simulink model "positioning_system"  (R2021a)
settings: Solver=ode45  StartTime=0.0  StopTime=2  RelTol=1e-3
values from neighbouring files (symbols this model uses):
  C = 0.33*(10^-6)    (= 3.3e-07)    [run_positioning_system.m]
  d = 1    [run_positioning_system.m]
  Km = 5*(10^-3)    (= 0.005)    [run_positioning_system.m]
  Ks = 52.5    [run_positioning_system.m]
  P = 60000    [run_positioning_system.m]
  R = 10000    [run_positioning_system.m]
settings Model: Creator=sujit  LastModifiedBy=cop20skj
settings SolverCC: AlgebraicLoopSolver=TrustRegion
settings DataIOCC: ReturnWorkspaceOutputs=off
settings DebuggingCC: SFMachineParentedDataDiag=warning

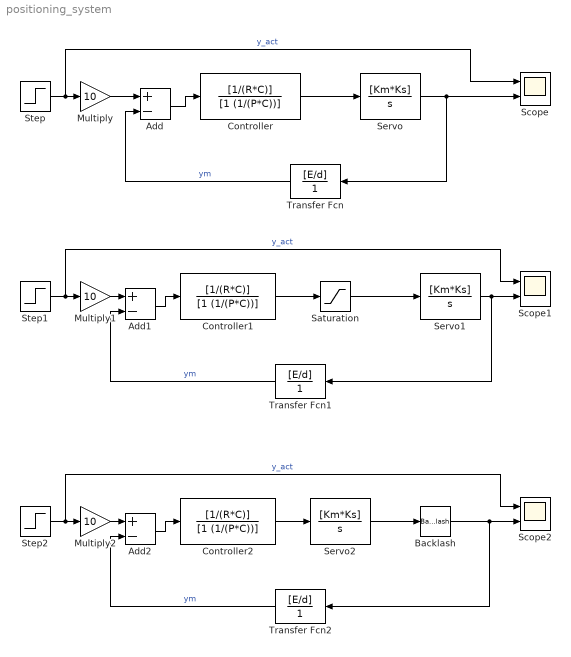
== system positioning_system ==
  Add : Sum  Inputs=+-
  Add1 : Sum  Inputs=+-
  Add2 : Sum  Inputs=+-
  Backlash : Backlash
  Controller : TransferFcn  Numerator=[1/(R*C)]  Denominator=[1 (1/(P*C))]
  Controller1 : TransferFcn  Numerator=[1/(R*C)]  Denominator=[1 (1/(P*C))]
  Controller2 : TransferFcn  Numerator=[1/(R*C)]  Denominator=[1 (1/(P*C))]
  Multiply : Gain  Gain=10
  Multiply1 : Gain  Gain=10
  Multiply2 : Gain  Gain=10
  Saturation : Saturate  UpperLimit=10  LowerLimit=-10
  Scope : Scope  NumInputPorts=2
  Scope1 : Scope  NumInputPorts=2
  Scope2 : Scope  NumInputPorts=2
  Servo : TransferFcn  Numerator=[Km*Ks]  Denominator=[1 0]
  Servo1 : TransferFcn  Numerator=[Km*Ks]  Denominator=[1 0]
  Servo2 : TransferFcn  Numerator=[Km*Ks]  Denominator=[1 0]
  Step : Step  SampleTime=0
  Step1 : Step  SampleTime=0
  Step2 : Step  SampleTime=0
  Transfer Fcn : TransferFcn  Numerator=[E/d]  Denominator=[1]
  Transfer Fcn1 : TransferFcn  Numerator=[E/d]  Denominator=[1]
  Transfer Fcn2 : TransferFcn  Numerator=[E/d]  Denominator=[1]
  wires:
  Multiply/1 -> Add/1
  Add/1 -> Controller/1
  Transfer Fcn/1 -> Add/2  "ym"
  Controller/1 -> Servo/1
  Servo/1 -> Scope/2, Transfer Fcn/1
  Step/1 -> Scope/1, Multiply/1  "y_act"
  Transfer Fcn1/1 -> Add1/2  "ym"
  Step1/1 -> Scope1/1, Multiply1/1  "y_act"
  Servo1/1 -> Scope1/2, Transfer Fcn1/1
  Add1/1 -> Controller1/1
  Multiply1/1 -> Add1/1
  Controller1/1 -> Saturation/1
  Saturation/1 -> Servo1/1
  Multiply2/1 -> Add2/1
  Add2/1 -> Controller2/1
  Transfer Fcn2/1 -> Add2/2  "ym"
  Step2/1 -> Scope2/1, Multiply2/1  "y_act"
  Controller2/1 -> Servo2/1
  Servo2/1 -> Backlash/1
  Backlash/1 -> Transfer Fcn2/1, Scope2/2
